simulink model "Tagani_Sugeno_Penduloinvertido_T7_Ejercicio3"  (R2024b)
settings: Solver=FixedStepAuto  StartTime=0.0  StopTime=5  FixedStep=0.001  RelTol=1e-3
values from neighbouring files (symbols this model uses):
  G_nl = [G1_nl G2_nl]    [Script_Tagani_Sugeno_T7.m]    (also in Script_Tagani_Sugeno_T7_Ejercicio3.m)
  G_ns = [G1_ns G2_ns]    [Script_Tagani_Sugeno_T7.m]    (also in Script_Tagani_Sugeno_T7_Ejercicio3.m)
  G_z = [G1_z G2_z]    [Script_Tagani_Sugeno_T7.m]    (also in Script_Tagani_Sugeno_T7_Ejercicio3.m)
  K_nl = place(A1, B1,p)    [Script_Tagani_Sugeno_T7.m]    (also in Script_Tagani_Sugeno_T7_Ejercicio3.m)
  K_ns = place(A2, B2,p)    [Script_Tagani_Sugeno_T7.m]    (also in Script_Tagani_Sugeno_T7_Ejercicio3.m)
  K_z = place(A3, B3,p)    [Script_Tagani_Sugeno_T7.m]    (also in Script_Tagani_Sugeno_T7_Ejercicio3.m)
  P_nl = [P11_nl P12_nl;P21_nl P22_nl]    [Script_Tagani_Sugeno_T7.m]    (also in Script_Tagani_Sugeno_T7_Ejercicio3.m = [P11_nl P12_nl;P21_nl P22_nl; P31_nl P32_nl;P41_nl P42_nl])
  P_ns = [P11_ns P12_ns;P21_ns P22_ns]    [Script_Tagani_Sugeno_T7.m]    (also in Script_Tagani_Sugeno_T7_Ejercicio3.m = [P11_ns P12_ns;P21_ns P22_ns; P31_ns P32_ns;P41_ns P42_ns])
  P_z = [P11_z P12_z;P21_z P22_z]    [Script_Tagani_Sugeno_T7.m]    (also in Script_Tagani_Sugeno_T7_Ejercicio3.m = [P11_z P12_z;P21_z P22_z; P31_z P32_z;P41_z P42_z])
settings Model: Creator=Usuario  LastModifiedBy=Lenovo

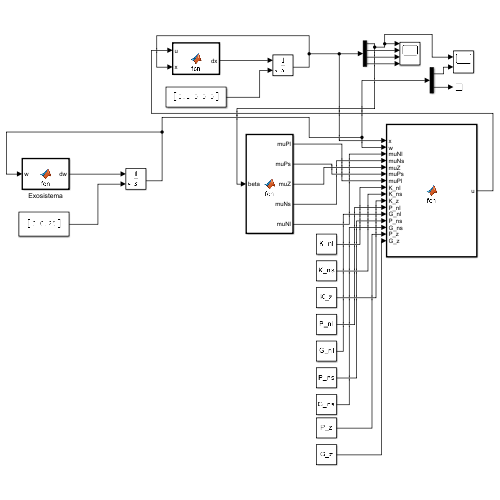
[thumbnail: Simulink's stored preview of the top-level diagram]
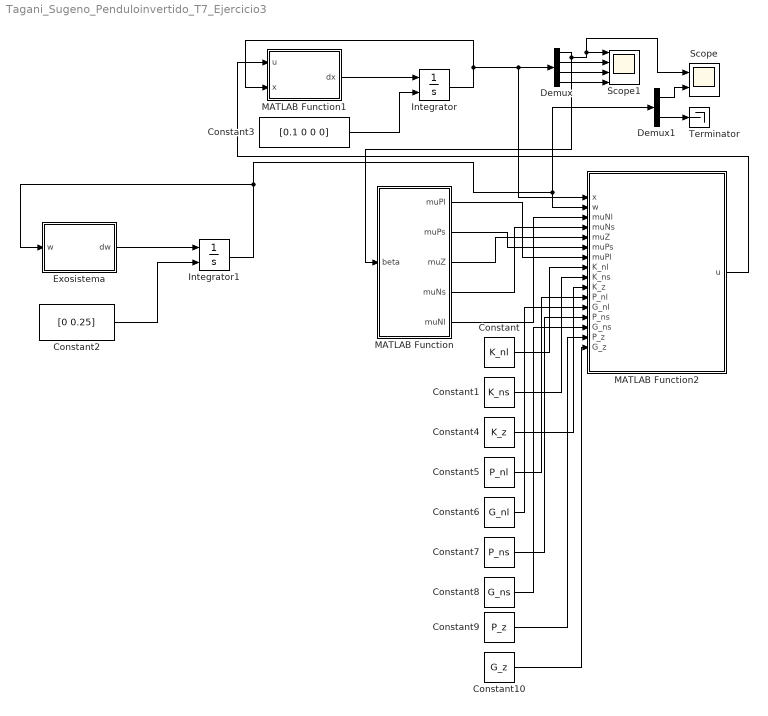
== system Tagani_Sugeno_Penduloinvertido_T7_Ejercicio3 ==
  Constant : Constant  Value=K_nl
  Constant1 : Constant  Value=K_ns
  Constant10 : Constant  Value=G_z
  Constant2 : Constant  Value=[0 0.25]
  Constant3 : Constant  Value=[0.1 0 0 0]
  Constant4 : Constant  Value=K_z
  Constant5 : Constant  Value=P_nl
  Constant6 : Constant  Value=G_nl
  Constant7 : Constant  Value=P_ns
  Constant8 : Constant  Value=G_ns
  Constant9 : Constant  Value=P_z
  Demux : Demux
  Demux1 : Demux  Outputs=2
  Exosistema : MATLAB Function  TreatAsAtomicUnit=on
  Integrator : Integrator  InitialConditionSource=external
  Integrator1 : Integrator  InitialConditionSource=external
  MATLAB Function : MATLAB Function  TreatAsAtomicUnit=on
  MATLAB Function1 : MATLAB Function  TreatAsAtomicUnit=on
  MATLAB Function2 : MATLAB Function  TreatAsAtomicUnit=on
  Scope : Scope  NumInputPorts=2
  Scope1 : Scope  NumInputPorts=4
  Terminator : Terminator
  wires:
  MATLAB Function/3(muZ) -> MATLAB Function2/5(muZ)
  MATLAB Function/5(muNl) -> MATLAB Function2/3(muNl)
  MATLAB Function/4(muNs) -> MATLAB Function2/4(muNs)
  MATLAB Function/2(muPs) -> MATLAB Function2/6(muPs)
  MATLAB Function/1(muPl) -> MATLAB Function2/7(muPl)
  MATLAB Function1/1(dx) -> Integrator/1
  Constant/1 -> MATLAB Function2/8(K_nl)
  Constant1/1 -> MATLAB Function2/9(K_ns)
  Exosistema/1(dw) -> Integrator1/1
  Constant2/1 -> Integrator1/2
  Integrator1/1 -> Exosistema/1(w), Demux1/1, MATLAB Function2/2(w)
  Constant3/1 -> Integrator/2
  Integrator/1 -> MATLAB Function2/1(x), Demux/1, MATLAB Function1/2(x)
  MATLAB Function2/1(u) -> MATLAB Function1/1(u)
  Demux1/2 -> Terminator/1
  Demux/1 -> MATLAB Function/1(beta), Scope/1, Scope1/1
  Demux/2 -> Scope1/2
  Demux1/1 -> Scope/2
  Constant4/1 -> MATLAB Function2/10(K_z)
  Constant5/1 -> MATLAB Function2/11(P_nl)
  Constant6/1 -> MATLAB Function2/12(G_nl)
  Constant7/1 -> MATLAB Function2/13(P_ns)
  Constant8/1 -> MATLAB Function2/14(G_ns)
  Constant9/1 -> MATLAB Function2/15(P_z)
  Constant10/1 -> MATLAB Function2/16(G_z)
  Demux/3 -> Scope1/3
  Demux/4 -> Scope1/4

== matlab function Tagani_Sugeno_Penduloinvertido_T7_Ejercicio3/MATLAB Function1 ==
  data: dx output; u input; x input
function dx  = fcn(u,x)

Rm=1.9;
Km=0.104;
Kg=0.055;
J=0.003; l1=0.12; l2=0.75; g=9.81; m2=0.50;
p1=(Kg*Km)/Rm;
p2=(Kg*Kg*Km*Km)/Rm;
x1=x(1);
x2=x(2);
x3=x(3);
x4=x(4);
dx1=x2;
dx2=((m2*l1^2 + J)*m2*l2*g*sin(x1)-m2*l1*l2*cos(x1)*(p1*u-p2*x4+m2*l1*l2*sin(x1)*x2*x4))/((m2*l1^2+J)*m2*l2^2-(m2*l1*l2*cos(x1))^2);
dx3=x4;
dx4=((m2*l2^2)*(p1*u-p2*x4 + m2*l1*l2*sin(x1)*x2*x4)-m2*l1*l2*cos(x1)*(m2*l2*g*sin(x1)))/((m2*l1^2+J)*m2*l2^2-(m2*l1*l2*cos(x1))^2);


dx = [dx1;dx2;dx3;dx4];

== matlab function Tagani_Sugeno_Penduloinvertido_T7_Ejercicio3/MATLAB Function ==
  data: muPl output; muPs output; muZ output; muNs output; muNl output; beta input
function [muPl, muPs, muZ, muNs, muNl] = fcn(beta)

% Para μ Positivo Large
if beta <= 7.5
    muPl = 0;
elseif beta > 7.5 && beta <= 15
    muPl = (beta - 7.5)/7.5;
else
    muPl = 1;
end

% Para μ Positivo Small
if beta <= 0
    muPs = 0;
elseif beta > 0 && beta <= 7.5
    muPs = beta/7.5;
elseif beta > 7.5 && beta <= 15
    muPs = (15 - beta)/7.5;
else
    muPs = 0;
end
%  Para μ Zero
if beta <= -7.5
    muZ = 0;
elseif beta > -7.5 && beta <= 0
    muZ = (beta + 7.5)/7.5;
elseif beta > 0 && beta <= 7.5
    muZ = (7.5 - beta)/7.5;
else
    muZ = 0;
end
% Para μ Negativo Small
if beta <= -15
    muNs = 0;
elseif beta > -15 && beta <= -7.5
    muNs = (beta + 15)/7.5;
elseif beta > -7.5 && beta <= 0
    muNs = -beta/7.5;
else
    muNs = 0;
end
% Para μ Negativo Large
if beta <= -15
    muNl = 1;
elseif beta > -15 && beta <= -7.5
    muNl = (-7.5 - beta)/7.5;
else
    muNl = 0;
end

end

== matlab function Tagani_Sugeno_Penduloinvertido_T7_Ejercicio3/MATLAB Function2 ==
  data: x input; u output; w input; muNl input; muNs input; muZ input; muPs input; muPl input; K_nl input; K_ns input; K_z input; P_nl input; G_nl input; P_ns input; G_ns input; P_z input; G_z input
function u = fcn(x, w, muNl, muNs, muZ, muPs, muPl, K_nl, K_ns, K_z, P_nl,G_nl,P_ns,G_ns,P_z,G_z)

%% 15 y 15
P_nl= [P_nl(1,1) P_nl(1,2);P_nl(2,1) P_nl(2,2);P_nl(3,1) P_nl(3,2);P_nl(4,1) P_nl(4,2)];
G_nl=[G_nl(1) G_nl(2)];
K_nl=[K_nl(1) K_nl(2) K_nl(3) K_nl(4)];
u_nl= -K_nl*x + (G_nl - K_nl*P_nl)*w;
u_pl=u_nl;

%% -7.5 y 7.5
P_ns= [P_ns(1,1) P_ns(1,2);P_ns(2,1) P_ns(2,2);P_ns(3,1) P_ns(3,2);P_ns(4,1) P_ns(4,2)];
G_ns=[G_ns(1) G_ns(2)];
K_ns=[K_ns(1) K_ns(2) K_ns(3) K_ns(4)];
u_ns= -K_ns*x + (G_ns - K_ns*P_ns)*w;
u_ps=u_ns;
%% 0
P_z= [P_z(1,1) P_z(1,2);P_z(2,1) P_z(2,2);P_z(3,1) P_z(3,2);P_z(4,1) P_z(4,2)];
G_z=[G_z(1) G_z(2)];
K_z=[K_z(1) K_z(2) K_z(3) K_z(4)];
u_z= -K_z*x + (G_z - K_z*P_z)*w;

%% Defusificacion
u=(u_nl*muNl + u_ns*muNs + u_z*muZ + u_ps*muPs + u_pl*muPl)/(muNl+ muNs+ muZ+ muPs+ muPl);

== matlab function Tagani_Sugeno_Penduloinvertido_T7_Ejercicio3/Exosistema ==
  data: w input; dw output
function dw = fcn(w)

dw=[0 10; -10 0]*w;
